simulink model "probm3"  (R2020a)
settings: Solver=VariableStepAuto  StartTime=0.0  StopTime=10.0  MaxStep=0.01  RelTol=1e-3
settings Model: Creator=DELL  LastModifiedBy=DELL

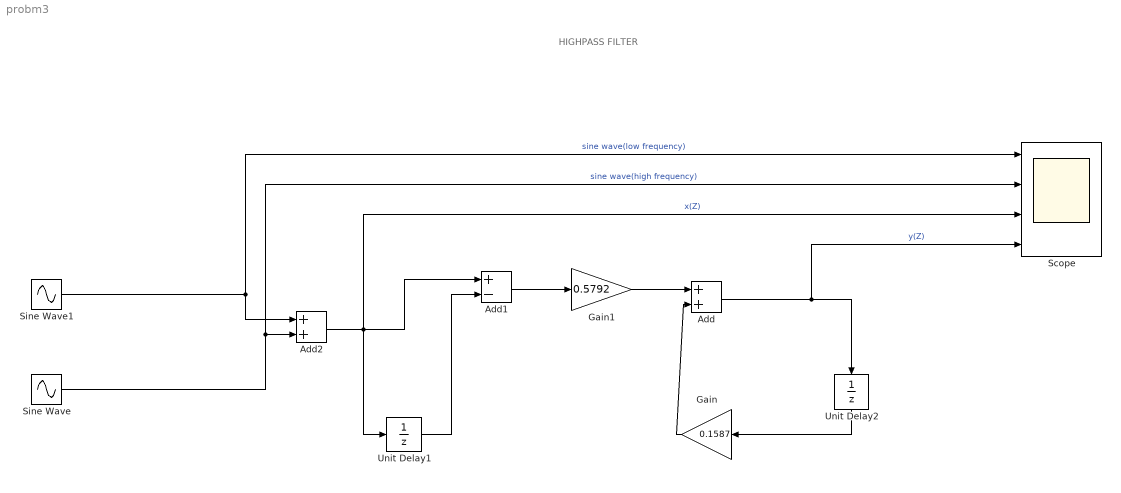
== system probm3 ==
  note: HIGHPASS FILTER
  Add : Sum
  Add1 : Sum  Inputs=+-
  Add2 : Sum
  Gain : Gain  Gain=0.1587
  Gain1 : Gain  Gain=0.5792
  Scope : Scope  NumInputPorts=4
  Sine Wave : Sin  Frequency=1800  SampleTime=0
  Sine Wave1 : Sin  Frequency=400  SampleTime=0
  Unit Delay1 : UnitDelay  SampleTime=-1  HasFrameUpgradeWarning=on
  Unit Delay2 : UnitDelay  SampleTime=-1  HasFrameUpgradeWarning=on
  wires:
  Add/1 -> Unit Delay2/1, Scope/4  "y(Z)"
  Unit Delay1/1 -> Add1/2
  Gain1/1 -> Add/1
  Gain/1 -> Add/2
  Sine Wave/1 -> Scope/2, Add2/2  "sine wave(high frequency)"
  Unit Delay2/1 -> Gain/1
  Add1/1 -> Gain1/1
  Sine Wave1/1 -> Add2/1, Scope/1  "sine wave(low frequency)"
  Add2/1 -> Scope/3, Unit Delay1/1, Add1/1  "x(Z)"
